simulink model "Mip_Balance_Demo_Multi_Rate"  (R2018b)
settings: Solver=FixedStepAuto  StartTime=0.0  StopTime=inf  RelTol=1e-3
undefined symbols (not defined in the file): DiscIntNeverNeededParam
libraries: simulink x2, bbblueSensorLib x2, bbblueActuatorLib x2, bbblueBasicLib x2, simulink_extras x1
settings Model: SimulationMode=external  Creator=ktalke  LastModifiedBy=ktalke
settings SolverCC: PositivePriorityOrder=on  AutoInsertRateTranBlk=on
settings OptimizationCC: EnhancedBackFolding=on  PassReuseOutputArgsAs=Individual arguments  MaxStackSize=64  OptimizeBlockOrder=speed  DifferentSizesBufferReuse=on  OptimizationCustomize=off
settings DebuggingCC: ParameterTunabilityLossMsg=error  LibraryContextMissingDiagnostic=none
settings HardwareCC: ProdBitPerPointer=32  ProdBitPerSizeT=32  ProdBitPerPtrDiffT=32  ProdLargestAtomicInteger=Long  ProdLargestAtomicFloat=Double  ProdWordSize=32  ProdHWDeviceType=ARM Compatible->ARM Cortex
settings SFSimCC: SimUseLocalCustomCode=off  MATLABDynamicMemAlloc=off
settings RTWCC: SystemTargetFile=ert.tlc  HardwareBoard=BeagleBone Blue  TLCOptions="-aInlineSetEventsForThisBaseRateFcn=TLC_FALSE -aSuppressMultiTaskScheduler=TLC_FALSE  -aRateBasedStepFcn=0"  TemplateMakefile=ert_default_tmf  RTWUseLocalCustomCode=off  Toolchain=GNU GCC BeagleBone Blue  IncludeHyperlinkInReport=on
settings CodeAppCC: ForceParamTrailComments=on  IgnoreCustomStorageClasses=off  OperatorAnnotations=on  SimulinkDataObjDesc=on  SFDataObjDesc=on  InsertBlockDesc=on
settings ERTTargetCC: SupportVariableSizeSignals=on

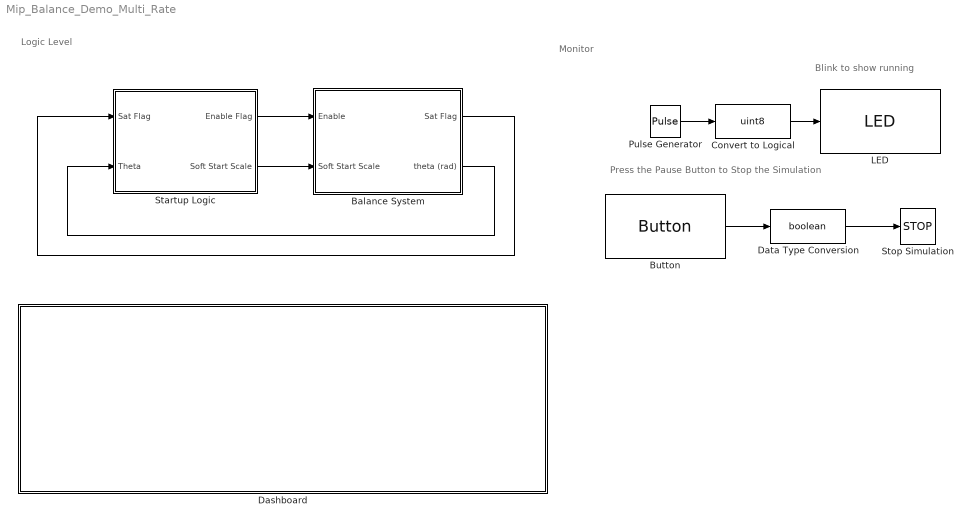
== system Mip_Balance_Demo_Multi_Rate ==
  note: Press the Pause Button to Stop the Simulation
  note: Logic Level
  note: Monitor
  note: Blink to show running
  Balance System : Subsystem  TreatAsAtomicUnit=on
  Button : bbblueBasicLib/Button  Button=Pause  SampleTime=0.1  SimulateUsing=Code generation
      settings: SourceProductName=Simulink Coder Support Package for BeagleBone Blue Hardware
  Convert to Logical : DataTypeConversion  OutDataTypeStr=uint8
  Dashboard : Subsystem
  Data Type Conversion : DataTypeConversion  OutDataTypeStr=boolean
  LED : bbblueBasicLib/LED  LED=Green
      settings: SourceProductName=Simulink Coder Support Package for BeagleBone Blue Hardware
  Pulse Generator : DiscretePulseGenerator  Period=10  PulseWidth=5  SampleTime=0.1
  Startup Logic : Subsystem
  Stop Simulation : Stop
  wires:
  Button/1 -> Data Type Conversion/1
  Startup Logic/2(Soft Start Scale) -> Balance System/2(Soft Start Scale)
  Pulse Generator/1 -> Convert to Logical/1
  Balance System/1(Sat Flag) -> Startup Logic/1(Sat Flag)
  Balance System/2(theta (rad)) -> Startup Logic/2(Theta)
  Data Type Conversion/1 -> Stop Simulation/1
  Startup Logic/1(Enable Flag) -> Balance System/1(Enable)
  Convert to Logical/1 -> LED/1

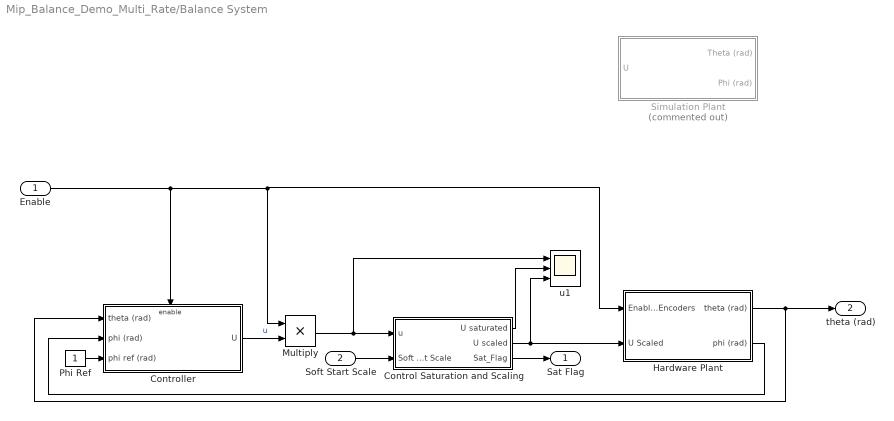
== system Mip_Balance_Demo_Multi_Rate/Balance System ==
  Enable : Inport
  Soft Start Scale : Inport  Port=2
  Control Saturation and Scaling : Subsystem
  Controller : Subsystem
  Hardware Plant : Subsystem
  Multiply : Product
  Phi Ref : Constant
  Simulation Plant : Subsystem  Commented=on
  u1 : Scope  NumInputPorts=3
  Sat Flag : Outport
  theta (rad) : Outport  Port=2
  wires:
  Phi Ref/1 -> Controller/3(phi ref (rad))
  Control Saturation and Scaling/1(U saturated) -> u1/2
  Control Saturation and Scaling/2(U scaled) -> Hardware Plant/2(U Scaled), u1/3
  Control Saturation and Scaling/3(Sat_Flag) -> Sat Flag/1
  Soft Start Scale/1 -> Control Saturation and Scaling/2(Soft Start Scale)
  Enable/1 -> Controller/Enable, Hardware Plant/1(Enable Encoders), Multiply/1
  Hardware Plant/1(theta (rad)) -> Controller/1(theta (rad)), theta (rad)/1
  Controller/1(U) -> Multiply/2  "u"
  Multiply/1 -> u1/1, Control Saturation and Scaling/1(u)
  Hardware Plant/2(phi (rad)) -> Controller/2(phi (rad))

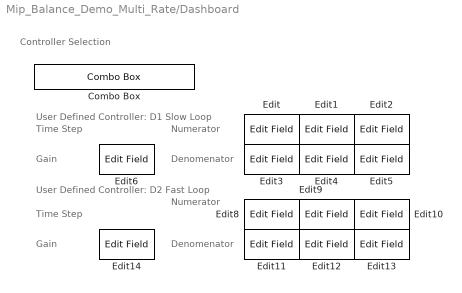
== system Mip_Balance_Demo_Multi_Rate/Dashboard ==
  note: Time Step
  note: Gain
  note: User Defined Controller: D1 Slow Loop
  note: Numerator
  note: Controller Selection
  note: Denomenator
  note: Numerator
  note: Denomenator
  note: Time Step
  note: User Defined Controller: D2 Fast Loop
  note: Gain
  Combo Box : ComboBox  WebBlockId=279  LabelPosition=Hide  SelectedLabel=200hz/20hz
      settings: Values={{'200 hz/200hz', '100hz/100hz', '100hz/50hz', '200hz/20hz', 'User Defined'}, [0 1 2 3 4]}
  Edit : EditField  WebBlockId=307  LabelPosition=Hide  ShowInitialText=on  Alignment=Center
  Edit1 : EditField  WebBlockId=313  LabelPosition=Hide  ShowInitialText=on  Alignment=Center
  Edit10 : EditField  WebBlockId=353  LabelPosition=Hide  ShowInitialText=on  Alignment=Center
  Edit11 : EditField  WebBlockId=354  LabelPosition=Hide  ShowInitialText=on  Alignment=Center
  Edit12 : EditField  WebBlockId=355  LabelPosition=Hide  ShowInitialText=on  Alignment=Center
  Edit13 : EditField  WebBlockId=356  LabelPosition=Hide  ShowInitialText=on  Alignment=Center
  Edit14 : EditField  WebBlockId=357  LabelPosition=Hide  ShowInitialText=on  Alignment=Center
  Edit2 : EditField  WebBlockId=314  LabelPosition=Hide  ShowInitialText=on  Alignment=Center
  Edit3 : EditField  WebBlockId=315  LabelPosition=Hide  ShowInitialText=on  Alignment=Center
  Edit4 : EditField  WebBlockId=316  LabelPosition=Hide  ShowInitialText=on  Alignment=Center
  Edit5 : EditField  WebBlockId=317  LabelPosition=Hide  ShowInitialText=on  Alignment=Center
  Edit6 : EditField  WebBlockId=337  LabelPosition=Hide  ShowInitialText=on  Alignment=Center
  Edit8 : EditField  WebBlockId=351  LabelPosition=Hide  ShowInitialText=on  Alignment=Center
  Edit9 : EditField  WebBlockId=352  LabelPosition=Hide  ShowInitialText=on  Alignment=Center

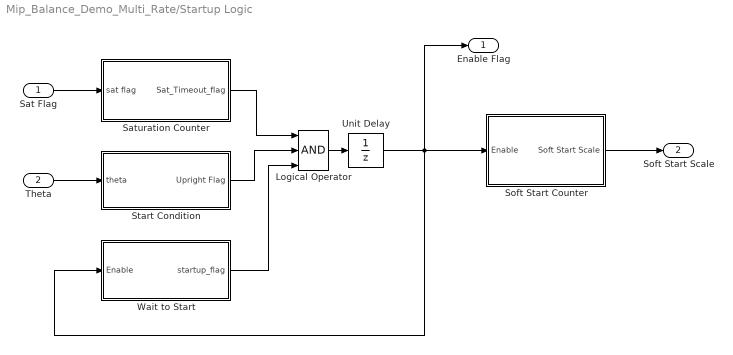
== system Mip_Balance_Demo_Multi_Rate/Startup Logic ==
  Sat Flag : Inport
  Theta : Inport  Port=2
  Logical Operator : Logic  Inputs=3  AllPortsSameDT=off  OutDataTypeStr=boolean
  Saturation Counter : Subsystem
  "Soft Start Counter " : Subsystem
  Start Condition : Subsystem
  Unit Delay : UnitDelay  SampleTime=-1
  Wait to Start : Subsystem
  Enable Flag : Outport
  Soft Start Scale : Outport  Port=2
  wires:
  Wait to Start/1(startup_flag) -> Logical Operator/3
  Logical Operator/1 -> Unit Delay/1
  Start Condition/1(Upright Flag) -> Logical Operator/2
  Saturation Counter/1(Sat_Timeout_flag) -> Logical Operator/1
  "Soft Start Counter "/1(Soft Start Scale) -> Soft Start Scale/1
  Sat Flag/1 -> Saturation Counter/1(sat flag)
  Theta/1 -> Start Condition/1(theta)
  Unit Delay/1 -> Enable Flag/1, "Soft Start Counter "/1(Enable), Wait to Start/1(Enable)

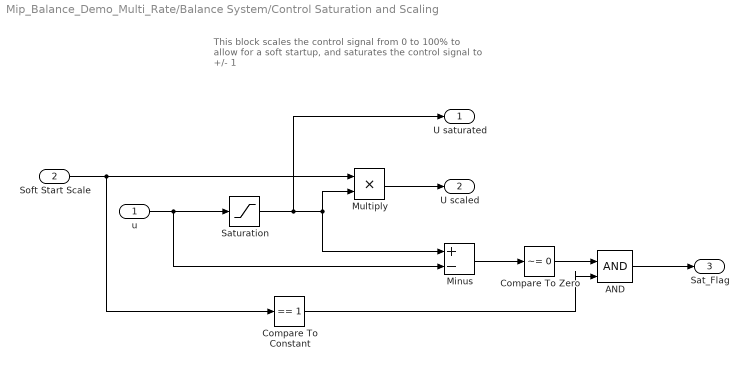
== system Mip_Balance_Demo_Multi_Rate/Balance System/Control Saturation and Scaling ==
  note: This block scales the control signal from 0 to 100% to allow for a soft startup, and saturates the control signal to +/- 1
  u : Inport
  Soft Start Scale : Inport  Port=2
  AND : Logic  IconShape=distinctive  AllPortsSameDT=off  OutDataTypeStr=boolean
  Compare To Constant : simulink/Logic and Bit Operations/Compare To Constant  relop===  const=1  OutDataTypeStr=boolean
  Compare To Zero : simulink/Logic and Bit Operations/Compare To Zero  relop=~=  OutDataTypeStr=boolean
  Minus : Sum  Inputs=+-
  Multiply : Product
  Saturation : Saturate  UpperLimit=1  LowerLimit=-1
  U saturated : Outport
  U scaled : Outport  Port=2  OutDataTypeStr=double  PortDimensions=[1 1]  SampleTime=[0.01,0]
  Sat_Flag : Outport  Port=3
  wires:
  u/1 -> Minus/2, Saturation/1
  Minus/1 -> Compare To Zero/1
  Soft Start Scale/1 -> Compare To Constant/1, Multiply/1
  Multiply/1 -> U scaled/1
  Saturation/1 -> U saturated/1, Minus/1, Multiply/2
  Compare To Zero/1 -> AND/1
  Compare To Constant/1 -> AND/2
  AND/1 -> Sat_Flag/1

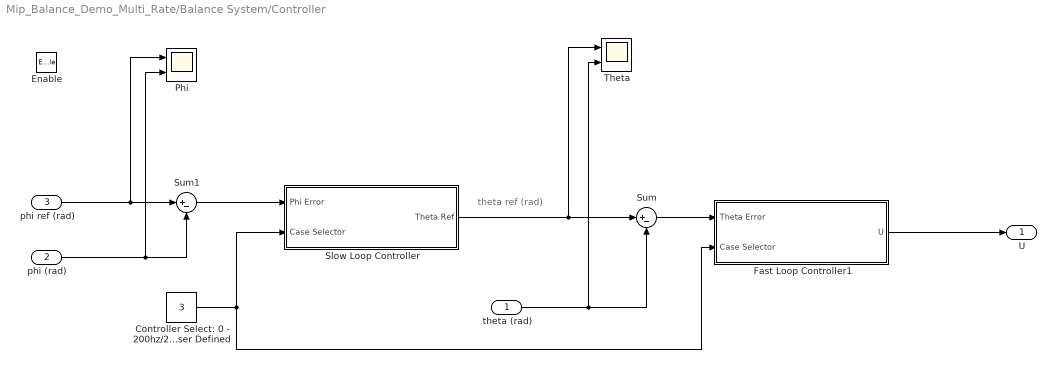
== system Mip_Balance_Demo_Multi_Rate/Balance System/Controller ==
  note: theta ref (rad)
  theta (rad) : Inport
  phi (rad) : Inport  Port=2
  phi ref (rad) : Inport  Port=3
  Enable : EnablePort  StatesWhenEnabling=reset  PropagateVarSize=During execution
  Controller Select: 0 - 200hz/200hz 1 - 100hz/100hz 2 - 100hz/50hz 3 - 200hz/20hz 4 - User Defined : Constant  Value=3
  Fast Loop Controller1 : Subsystem
  Phi : Scope  NumInputPorts=2
  Slow Loop Controller : Subsystem
  Sum : Sum  Inputs=|+-
  Sum1 : Sum  Inputs=|+-
  Theta : Scope  NumInputPorts=2
  U : Outport
  wires:
  phi ref (rad)/1 -> Phi/1, Sum1/1
  theta (rad)/1 -> Theta/2, Sum/2
  phi (rad)/1 -> Sum1/2, Phi/2
  Sum1/1 -> Slow Loop Controller/1(Phi Error)
  Slow Loop Controller/1(Theta Ref) -> Theta/1, Sum/1
  Controller Select: 0 - 200hz/200hz 1 - 100hz/100hz 2 - 100hz/50hz 3 - 200hz/20hz 4 - User Defined/1 -> Fast Loop Controller1/2(Case Selector), Slow Loop Controller/2(Case Selector)
  Sum/1 -> Fast Loop Controller1/1(Theta Error)
  Fast Loop Controller1/1(U) -> U/1

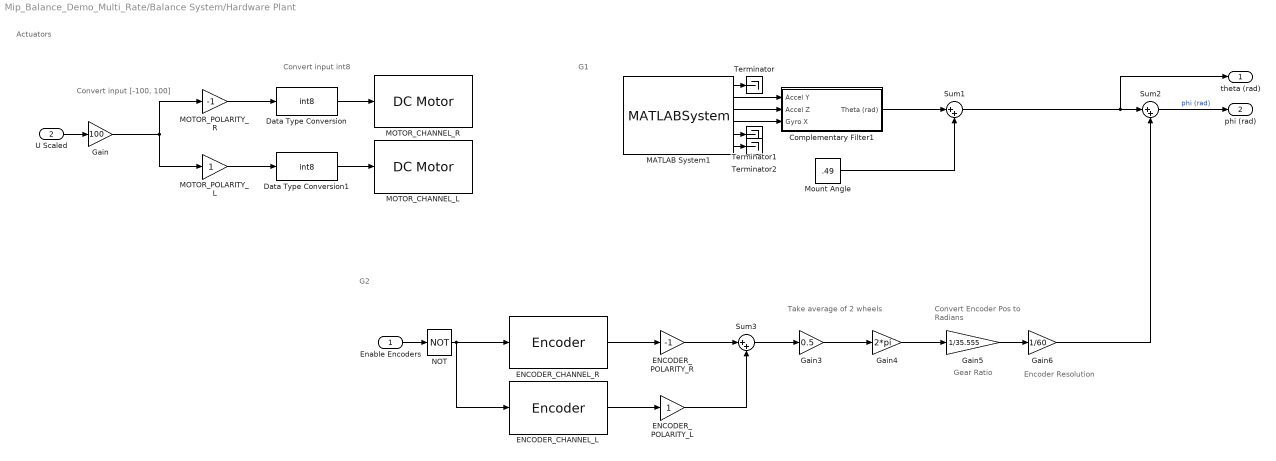
== system Mip_Balance_Demo_Multi_Rate/Balance System/Hardware Plant ==
  note: G2
  note: G1
  note: Actuators
  note: Convert input
      | [-100, 100]
  note: Convert input
      | int8
  note: Gear Ratio
  note: Encoder
      | Resolution
  note: Convert Encoder Pos
      | to Radians
  note: Take average
      | of 2 wheels
  Enable Encoders : Inport
  U Scaled : Inport  Port=2
  Complementary Filter1 : Subsystem
  Data Type Conversion : DataTypeConversion  OutDataTypeStr=int8  SaturateOnIntegerOverflow=on  RndMeth=Zero
  Data Type Conversion1 : DataTypeConversion  OutDataTypeStr=int8  SaturateOnIntegerOverflow=on  RndMeth=Zero
  ENCODER_CHANNEL_L : bbblueSensorLib/Encoder  Channel=3  Mode=Reset by external signal  SampleTime=0.005  SimulateUsing=Code generation
      settings: SourceProductName=Simulink Coder Support Package for BeagleBone Blue Hardware
  ENCODER_CHANNEL_R : bbblueSensorLib/Encoder  Channel=2  Mode=Reset by external signal  SampleTime=0.005  SimulateUsing=Code generation
      settings: SourceProductName=Simulink Coder Support Package for BeagleBone Blue Hardware
  ENCODER_POLARITY_L : Gain
  ENCODER_POLARITY_R : Gain  Gain=-1
  Gain : Gain  Gain=100
  Gain3 : Gain  Gain=0.5  OutDataTypeStr=double
  Gain4 : Gain  Gain=2*pi
  Gain5 : Gain  Gain=1/35.555
  Gain6 : Gain  Gain=1/60
  MATLAB System1 : MATLABSystem  System=beagleboneblue.fccr_bbblueIMU  SampleTime=0.005
      mask Type: beagleboneblue.fccr_bbblueIMU
      mask Display:
      | color('white');
      | plot([100,100,100,100]*1,[100,100,100,100]*1);
      | plot([100,100,100,100]*0,[100,100,100,100]*0);
      | color('blue');
      | text(100, 92, ' BB BLUE ', 'horizontalAlignment', 'right');
      | color('black');
      | text(52,52,' IMU','horizontalAlignment','center');
      | color('black');
  MOTOR_CHANNEL_L : bbblueActuatorLib/DC Motor  index=3  stopaction=Free Spin  SimulateUsing=Code generation
      settings: SourceProductName=Simulink Coder Support Package for BeagleBone Blue Hardware
  MOTOR_CHANNEL_R : bbblueActuatorLib/DC Motor  index=2  stopaction=Free Spin  SimulateUsing=Code generation
      settings: SourceProductName=Simulink Coder Support Package for BeagleBone Blue Hardware
  MOTOR_POLARITY_L : Gain
  MOTOR_POLARITY_R : Gain  Gain=-1
  Mount Angle : Constant  Value=.49
  NOT : Logic  Operator=NOT  IconShape=distinctive  AllPortsSameDT=off  OutDataTypeStr=boolean
  Sum1 : Sum  Inputs=|++
  Sum2 : Sum  Inputs=|++
  Sum3 : Sum  Inputs=|++
  Terminator : Terminator
  Terminator1 : Terminator
  Terminator2 : Terminator
  theta (rad) : Outport
  phi (rad) : Outport  Port=2
  wires:
  Sum2/1 -> phi (rad)/1  "phi (rad)"
  Gain6/1 -> Sum2/2
  Data Type Conversion1/1 -> MOTOR_CHANNEL_L/1
  MOTOR_POLARITY_R/1 -> Data Type Conversion/1
  Data Type Conversion/1 -> MOTOR_CHANNEL_R/1
  U Scaled/1 -> Gain/1
  MOTOR_POLARITY_L/1 -> Data Type Conversion1/1
  Gain/1 -> MOTOR_POLARITY_R/1, MOTOR_POLARITY_L/1
  Sum1/1 -> theta (rad)/1, Sum2/1
  MATLAB System1/1 -> Terminator/1
  Mount Angle/1 -> Sum1/2
  MATLAB System1/6 -> Terminator2/1
  Complementary Filter1/1(Theta (rad)) -> Sum1/1
  MATLAB System1/5 -> Terminator1/1
  Enable Encoders/1 -> NOT/1
  Gain5/1 -> Gain6/1
  ENCODER_CHANNEL_R/1 -> ENCODER_POLARITY_R/1
  Sum3/1 -> Gain3/1
  ENCODER_POLARITY_R/1 -> Sum3/1
  NOT/1 -> ENCODER_CHANNEL_L/1, ENCODER_CHANNEL_R/1
  Gain4/1 -> Gain5/1
  ENCODER_CHANNEL_L/1 -> ENCODER_POLARITY_L/1
  ENCODER_POLARITY_L/1 -> Sum3/2
  Gain3/1 -> Gain4/1
  MATLAB System1/2 -> Complementary Filter1/1(Accel Y)
  MATLAB System1/3 -> Complementary Filter1/2(Accel Z)
  MATLAB System1/4 -> Complementary Filter1/3(Gyro X)

== system Mip_Balance_Demo_Multi_Rate/Balance System/Simulation Plant ==
  U : Inport
  G1 Transfer Function : TransferFcn  Numerator=-420.4  Denominator=[1 12.1 088.24 -963.6]
  G2 Transfer Function : TransferFcn  Numerator=[-0.0002636 0 113.4]  Denominator=[1 0 0]
  Theta (rad) : Outport
  Phi (rad) : Outport  Port=2
  wires:
  G2 Transfer Function/1 -> Phi (rad)/1
  U/1 -> G1 Transfer Function/1
  G1 Transfer Function/1 -> G2 Transfer Function/1, Theta (rad)/1

== system Mip_Balance_Demo_Multi_Rate/Startup Logic/Saturation Counter ==
  note: Saturation Detection Threshold:
      | This block checks how long the motor has been saturated, and generates a disable flag
  sat flag : Inport
  Discrete-Time Integrator : DiscreteIntegrator  ExternalReset=falling  SampleTime=-1  ICPrevOutput=DiscIntNeverNeededParam  ICPrevScaledInput=DiscIntNeverNeededParam
  Relational Operator : RelationalOperator  Operator=<  OutDataTypeStr=boolean  RndMeth=Simplest
  Sat Timeout : Constant  Value=.5
  Sat_Timeout_flag : Outport
  wires:
  Relational Operator/1 -> Sat_Timeout_flag/1
  Sat Timeout/1 -> Relational Operator/2
  Discrete-Time Integrator/1 -> Relational Operator/1
  sat flag/1 -> Discrete-Time Integrator/1, Discrete-Time Integrator/2

== system Mip_Balance_Demo_Multi_Rate/Startup Logic/Soft Start Counter  ==
  note: Soft Start Detection Threshold:
      | This block generates a signal to scale up the input from 0 to 100% for the specified soft start time
  Enable : Inport
  Data Type Conversion : DataTypeConversion  OutDataTypeStr=double
  Discrete-Time Integrator : DiscreteIntegrator  ExternalReset=rising  SampleTime=-1  ICPrevOutput=DiscIntNeverNeededParam  ICPrevScaledInput=DiscIntNeverNeededParam
  Limits : Product  Inputs=*/
  Saturation : Saturate  UpperLimit=1  LowerLimit=0
  Soft Start Time1 : Constant  Value=.9
  Soft Start Scale : Outport
  wires:
  Limits/1 -> Saturation/1
  Discrete-Time Integrator/1 -> Limits/1
  Soft Start Time1/1 -> Limits/2
  Enable/1 -> Data Type Conversion/1, Discrete-Time Integrator/2
  Saturation/1 -> Soft Start Scale/1
  Data Type Conversion/1 -> Discrete-Time Integrator/1

== system Mip_Balance_Demo_Multi_Rate/Startup Logic/Start Condition ==
  note: Upright Detection Threshold:
      | This block checks the angle theta to see if it near the stability point, and produces an enable flag
  theta : Inport
  Abs : Abs
  Relational Operator : RelationalOperator  OutDataTypeStr=boolean  RndMeth=Simplest
  Relational Operator1 : RelationalOperator  Operator=<  OutDataTypeStr=boolean  RndMeth=Simplest
  Start Angle : Constant  Value=.6
  Start Counter : DiscreteIntegrator  ExternalReset=falling  SampleTime=-1  RndMeth=Zero  SaturateOnIntegerOverflow=on  UpperSaturationLimit=100  LowerSaturationLimit=-100  ICPrevOutput=DiscIntNeverNeededParam  ICPrevScaledInput=DiscIntNeverNeededParam
  Start Timeout : Constant
  Upright Flag : Outport
  wires:
  theta/1 -> Abs/1
  Start Counter/1 -> Relational Operator/1
  Relational Operator/1 -> Upright Flag/1
  Abs/1 -> Relational Operator1/1
  Start Timeout/1 -> Relational Operator/2
  Relational Operator1/1 -> Start Counter/2, Start Counter/1
  Start Angle/1 -> Relational Operator1/2

== system Mip_Balance_Demo_Multi_Rate/Startup Logic/Wait to Start ==
  note: Startup Detection Threshold:
      | This block enforces a wait time before allowing any control to start. The purpose is to allow the complementary filter time to stabilize, and to give a break if any other disable flag was triggered.
  Enable : Inport
  Constant : Constant
  Relational Operator : RelationalOperator  OutDataTypeStr=boolean  RndMeth=Simplest
  Wait Counter : DiscreteIntegrator  ExternalReset=falling  SampleTime=-1  SaturateOnIntegerOverflow=on  ICPrevOutput=DiscIntNeverNeededParam  ICPrevScaledInput=DiscIntNeverNeededParam
  Wait to Start : Constant  Value=3
  startup_flag : Outport
  wires:
  Wait Counter/1 -> Relational Operator/1
  Constant/1 -> Wait Counter/1
  Wait to Start/1 -> Relational Operator/2
  Relational Operator/1 -> startup_flag/1
  Enable/1 -> Wait Counter/2

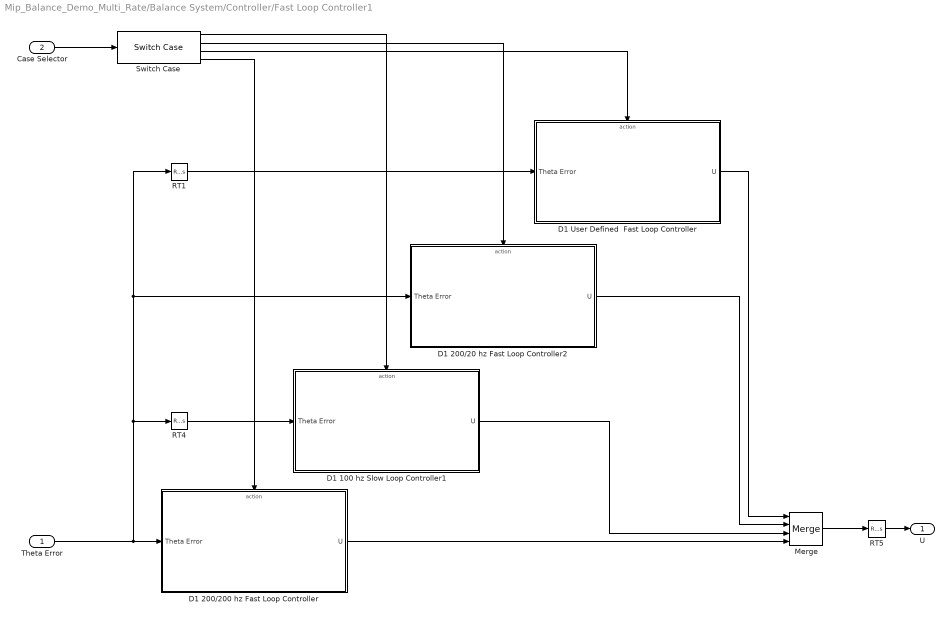
== system Mip_Balance_Demo_Multi_Rate/Balance System/Controller/Fast Loop Controller1 ==
  Theta Error : Inport
  Case Selector : Inport  Port=2
  D1 100 hz Slow Loop Controller1 : Subsystem  TreatAsAtomicUnit=on
  D1 200/20 hz Fast Loop Controller2 : Subsystem  TreatAsAtomicUnit=on
  D1 200/200 hz Fast Loop Controller : Subsystem  TreatAsAtomicUnit=on
  D1 User Defined  Fast Loop Controller : Subsystem  TreatAsAtomicUnit=on
  Merge : Merge  Inputs=4
  RT1 : RateTransition  OutPortSampleTime=0.005
  RT4 : RateTransition  OutPortSampleTime=0.01
  RT5 : RateTransition  OutPortSampleTime=0.005
  Switch Case : SwitchCase  CaseConditions={[1,2],3,4}
  U : Outport
  wires:
  Case Selector/1 -> Switch Case/1
  Theta Error/1 -> RT4/1, RT1/1, D1 200/20 hz Fast Loop Controller2/1(Theta Error), D1 200/200 hz Fast Loop Controller/1(Theta Error)
  Switch Case/4 -> D1 200/200 hz Fast Loop Controller/Action
  RT4/1 -> D1 100 hz Slow Loop Controller1/1(Theta Error)
  Merge/1 -> RT5/1
  RT5/1 -> U/1
  Switch Case/1 -> D1 100 hz Slow Loop Controller1/Action
  Switch Case/2 -> D1 200/20 hz Fast Loop Controller2/Action
  RT1/1 -> D1 User Defined  Fast Loop Controller/1(Theta Error)
  D1 User Defined  Fast Loop Controller/1(U) -> Merge/1
  D1 200/20 hz Fast Loop Controller2/1(U) -> Merge/2
  D1 100 hz Slow Loop Controller1/1(U) -> Merge/3
  D1 200/200 hz Fast Loop Controller/1(U) -> Merge/4
  Switch Case/3 -> D1 User Defined  Fast Loop Controller/Action

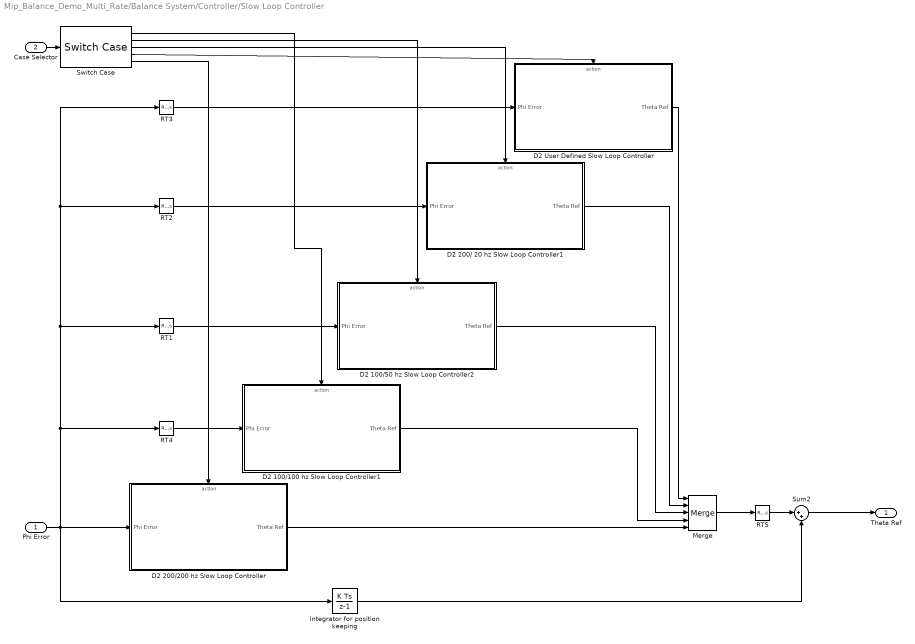
== system Mip_Balance_Demo_Multi_Rate/Balance System/Controller/Slow Loop Controller ==
  Phi Error : Inport
  Case Selector : Inport  Port=2
  D2 100/100 hz Slow Loop Controller1 : Subsystem  TreatAsAtomicUnit=on
  D2 100/50 hz Slow Loop Controller2 : Subsystem  TreatAsAtomicUnit=on
  "D2 200/ 20 hz Slow Loop Controller1 " : Subsystem  TreatAsAtomicUnit=on
  D2 200/200 hz Slow Loop Controller : Subsystem  TreatAsAtomicUnit=on
  D2 User Defined Slow Loop Controller : Subsystem  TreatAsAtomicUnit=on
  Integrator for position keeping : DiscreteIntegrator  gainval=.005  SampleTime=-1  ICPrevOutput=DiscIntNeverNeededParam  ICPrevScaledInput=DiscIntNeverNeededParam
  Merge : Merge  Inputs=5
  RT1 : RateTransition  OutPortSampleTime=0.02
  RT2 : RateTransition  OutPortSampleTime=0.05
  RT3 : RateTransition  OutPortSampleTimeMultiple=.1  OutPortSampleTime=0.01
  RT4 : RateTransition  OutPortSampleTime=0.01
  RT5 : RateTransition  OutPortSampleTime=0.005
  Sum2 : Sum  Inputs=|++
  Switch Case : SwitchCase  CaseConditions={1,2,3,4}
  Theta Ref : Outport
  wires:
  Case Selector/1 -> Switch Case/1
  Switch Case/5 -> D2 200/200 hz Slow Loop Controller/Action
  Switch Case/1 -> D2 100/100 hz Slow Loop Controller1/Action
  RT4/1 -> D2 100/100 hz Slow Loop Controller1/1(Phi Error)
  Merge/1 -> RT5/1
  Switch Case/2 -> D2 100/50 hz Slow Loop Controller2/Action
  Switch Case/3 -> "D2 200/ 20 hz Slow Loop Controller1 "/Action
  RT2/1 -> "D2 200/ 20 hz Slow Loop Controller1 "/1(Phi Error)
  RT1/1 -> D2 100/50 hz Slow Loop Controller2/1(Phi Error)
  Integrator for position keeping/1 -> Sum2/2
  Phi Error/1 -> Integrator for position keeping/1, RT3/1, RT2/1, RT1/1, RT4/1, D2 200/200 hz Slow Loop Controller/1(Phi Error)
  Sum2/1 -> Theta Ref/1
  RT5/1 -> Sum2/1
  D2 200/200 hz Slow Loop Controller/1(Theta Ref) -> Merge/5
  D2 100/100 hz Slow Loop Controller1/1(Theta Ref) -> Merge/4
  D2 100/50 hz Slow Loop Controller2/1(Theta Ref) -> Merge/3
  "D2 200/ 20 hz Slow Loop Controller1 "/1(Theta Ref) -> Merge/2
  RT3/1 -> D2 User Defined Slow Loop Controller/1(Phi Error)
  Switch Case/4 -> D2 User Defined Slow Loop Controller/Action
  D2 User Defined Slow Loop Controller/1(Theta Ref) -> Merge/1

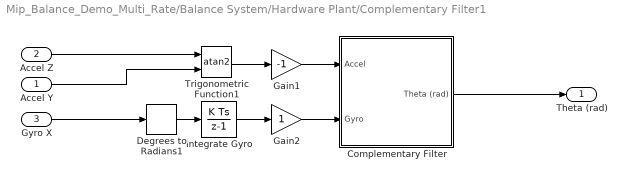
== system Mip_Balance_Demo_Multi_Rate/Balance System/Hardware Plant/Complementary Filter1 ==
  Accel Y : Inport
  Accel Z : Inport  Port=2
  Gyro X : Inport  Port=3
  Complementary Filter : Subsystem  mask(Complementary Filters){wc=.5, dt=.005}
      mask help:
      | dt - time step
      | wc - time constant
  Degrees to Radians1 : simulink_extras/Transformations/Degrees to Radians
  Gain1 : Gain  Gain=-1
  Gain2 : Gain
  Integrate Gyro : DiscreteIntegrator  SampleTime=-1  ICPrevOutput=DiscIntNeverNeededParam  ICPrevScaledInput=DiscIntNeverNeededParam
  Trigonometric Function1 : Trigonometry  Operator=atan2
  Theta (rad) : Outport
  wires:
  Complementary Filter/1(Theta (rad)) -> Theta (rad)/1
  Accel Z/1 -> Trigonometric Function1/1
  Gyro X/1 -> Degrees to Radians1/1
  Integrate Gyro/1 -> Gain2/1
  Degrees to Radians1/1 -> Integrate Gyro/1
  Accel Y/1 -> Trigonometric Function1/2
  Gain1/1 -> Complementary Filter/1(Accel)
  Trigonometric Function1/1 -> Gain1/1
  Gain2/1 -> Complementary Filter/2(Gyro)

== system Mip_Balance_Demo_Multi_Rate/Balance System/Controller/Fast Loop Controller1/D1 100 hz Slow Loop Controller1 ==
  Theta Error : Inport
  Action Port : ActionPort  ActionType=case
  D1 100hz Fast Loop Controller1 : DiscreteTransferFcn  Numerator=[-4.945, 8.862, -3.967]  Denominator=[1.000, -1.481, 0.4812]
  D1_GAIN1 : Gain  Gain=1.3
  U : Outport
  wires:
  D1 100hz Fast Loop Controller1/1 -> U/1
  D1_GAIN1/1 -> D1 100hz Fast Loop Controller1/1
  Theta Error/1 -> D1_GAIN1/1

== system Mip_Balance_Demo_Multi_Rate/Balance System/Controller/Fast Loop Controller1/D1 200//20 hz Fast Loop Controller2 ==
  Theta Error : Inport
  Action Port : ActionPort  ActionType=case
  D1 200hz/20hz Fast Loop Controller1 : DiscreteTransferFcn  Numerator=[-11.0745, 19.702, -8.7598]  Denominator=[1.000, -1.49756, 0.49756]
  D1_GAIN2 : Gain  Gain=.8
  U : Outport
  wires:
  D1 200hz/20hz Fast Loop Controller1/1 -> U/1
  D1_GAIN2/1 -> D1 200hz/20hz Fast Loop Controller1/1
  Theta Error/1 -> D1_GAIN2/1

== system Mip_Balance_Demo_Multi_Rate/Balance System/Controller/Fast Loop Controller1/D1 200//200 hz Fast Loop Controller ==
  Theta Error : Inport
  Action Port : ActionPort  ActionType=default
  D1 200hz/200hz Fast Loop Controller : DiscreteTransferFcn  Numerator=[-6.289, 11.91, -5.634]  Denominator=[1.000, -1.702, 0.7021]
  D1_GAIN : Gain  Gain=.8
  U : Outport
  wires:
  D1 200hz/200hz Fast Loop Controller/1 -> U/1
  D1_GAIN/1 -> D1 200hz/200hz Fast Loop Controller/1
  Theta Error/1 -> D1_GAIN/1

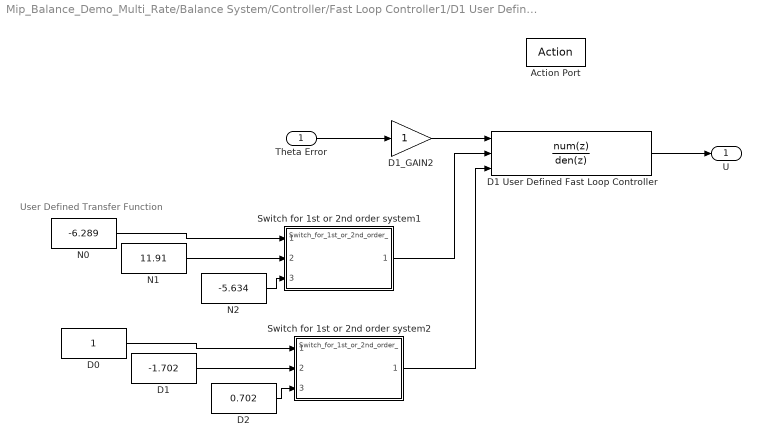
== system Mip_Balance_Demo_Multi_Rate/Balance System/Controller/Fast Loop Controller1/D1 User Defined  Fast Loop Controller ==
  note: User Defined Transfer Function
  Theta Error : Inport
  Action Port : ActionPort  ActionType=case
  D0 : Constant
  D1 : Constant  Value=-1.702
  D1 User Defined Fast Loop Controller : DiscreteTransferFcn  NumeratorSource=Input port  DenominatorSource=Input port  a0EqualsOne=on
      settings: InputPortMap=u0,p1,p3
  D1_GAIN2 : Gain
  D2 : Constant  Value=0.702
  N0 : Constant  Value=-6.289
  N1 : Constant  Value=11.91
  N2 : Constant  Value=-5.634
  Switch for 1st or 2nd order system1 : ModelReference  ModelNameDialog=Switch_for_1st_or_2nd_order_  SimulationMode=Normal  ModelReferenceVersion=1.140
  Switch for 1st or 2nd order system2 : ModelReference  ModelNameDialog=Switch_for_1st_or_2nd_order_  SimulationMode=Normal  ModelReferenceVersion=1.140
  U : Outport
  wires:
  D1 User Defined Fast Loop Controller/1 -> U/1
  D1_GAIN2/1 -> D1 User Defined Fast Loop Controller/1
  Theta Error/1 -> D1_GAIN2/1
  D2/1 -> Switch for 1st or 2nd order system2/3
  D0/1 -> Switch for 1st or 2nd order system2/1
  D1/1 -> Switch for 1st or 2nd order system2/2
  N0/1 -> Switch for 1st or 2nd order system1/1
  N2/1 -> Switch for 1st or 2nd order system1/3
  Switch for 1st or 2nd order system1/1 -> D1 User Defined Fast Loop Controller/2
  Switch for 1st or 2nd order system2/1 -> D1 User Defined Fast Loop Controller/3
  N1/1 -> Switch for 1st or 2nd order system1/2

== system Mip_Balance_Demo_Multi_Rate/Balance System/Controller/Slow Loop Controller/D2 100//100 hz Slow Loop Controller1 ==
  Phi Error : Inport
  Action Port : ActionPort  ActionType=case
  D2 100 hz Slow Loop Controller2 : DiscreteTransferFcn  Numerator="[0.28,  -0.5581,  0.2781]"  Denominator="[1.00000,  -1.86046,   0.86046]"
  D2_GAIN2 : Gain  Gain=.9
  Theta Ref : Outport
  wires:
  D2_GAIN2/1 -> D2 100 hz Slow Loop Controller2/1
  Phi Error/1 -> D2_GAIN2/1
  D2 100 hz Slow Loop Controller2/1 -> Theta Ref/1

== system Mip_Balance_Demo_Multi_Rate/Balance System/Controller/Slow Loop Controller/D2 100//50 hz Slow Loop Controller2 ==
  Phi Error : Inport
  Action Port : ActionPort  ActionType=case
  D2 50 hz SlowLoop Controller2 : DiscreteTransferFcn  Numerator="[0.2627,  -.5217, 0.259]"  Denominator="[1.00000,  -1.739, 0.7391]"
  D2_GAIN1 : Gain  Gain=.7
  Theta Ref : Outport
  wires:
  Phi Error/1 -> D2_GAIN1/1
  D2 50 hz SlowLoop Controller2/1 -> Theta Ref/1
  D2_GAIN1/1 -> D2 50 hz SlowLoop Controller2/1

== system Mip_Balance_Demo_Multi_Rate/Balance System/Controller/Slow Loop Controller/D2 200// 20 hz Slow Loop Controller1  ==
  Phi Error : Inport
  Action Port : ActionPort  ActionType=case
  D2 20 hz Slow Loop Controller2 : DiscreteTransferFcn  Numerator=[0.1636, -0.16289]  Denominator="[1.00000,  -.6326]"
  D2_GAIN3 : Gain  Gain=.7
  Theta Ref : Outport
  wires:
  D2 20 hz Slow Loop Controller2/1 -> Theta Ref/1
  D2_GAIN3/1 -> D2 20 hz Slow Loop Controller2/1
  Phi Error/1 -> D2_GAIN3/1

== system Mip_Balance_Demo_Multi_Rate/Balance System/Controller/Slow Loop Controller/D2 200//200 hz Slow Loop Controller ==
  Phi Error : Inport
  Action Port : ActionPort  ActionType=default
  D2 200 hz Slow Loop Controller1 : DiscreteTransferFcn  Numerator=[0.3858, -0.3858]  Denominator="[1.00000,  -.9277]"
  D2_GAIN : Gain  Gain=.7
  Theta Ref : Outport
  wires:
  D2 200 hz Slow Loop Controller1/1 -> Theta Ref/1
  Phi Error/1 -> D2_GAIN/1
  D2_GAIN/1 -> D2 200 hz Slow Loop Controller1/1

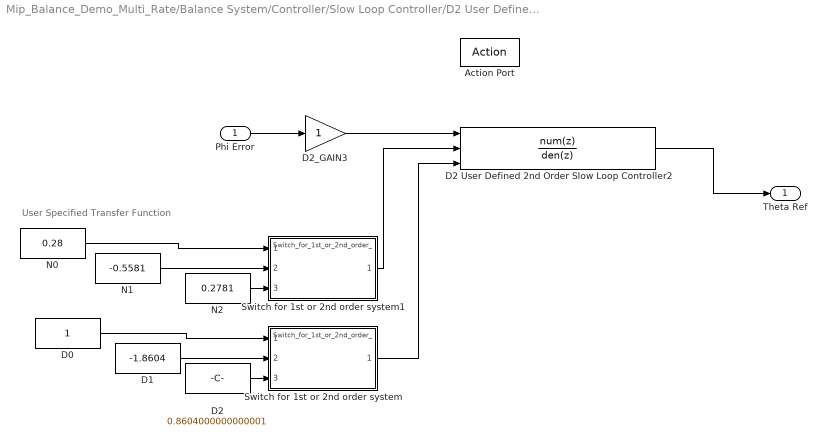
== system Mip_Balance_Demo_Multi_Rate/Balance System/Controller/Slow Loop Controller/D2 User Defined Slow Loop Controller ==
  note: User Specified Transfer Function
  Phi Error : Inport
  Action Port : ActionPort  ActionType=case
  D0 : Constant
  D1 : Constant  Value=-1.8604
  D2 : Constant  Value=0.8604000000000001
  D2 User Defined 2nd Order Slow Loop Controller2 : DiscreteTransferFcn  NumeratorSource=Input port  DenominatorSource=Input port  a0EqualsOne=on
      settings: InputPortMap=u0,p1,p3
  D2_GAIN3 : Gain
  N0 : Constant  Value=0.28
  N1 : Constant  Value=-0.5581
  N2 : Constant  Value=0.2781
  Switch for 1st or 2nd order system : ModelReference  ModelNameDialog=Switch_for_1st_or_2nd_order_  SimulationMode=Normal  ModelReferenceVersion=1.140
  Switch for 1st or 2nd order system1 : ModelReference  ModelNameDialog=Switch_for_1st_or_2nd_order_  SimulationMode=Normal  ModelReferenceVersion=1.140
  Theta Ref : Outport
  wires:
  D2_GAIN3/1 -> D2 User Defined 2nd Order Slow Loop Controller2/1
  Phi Error/1 -> D2_GAIN3/1
  N0/1 -> Switch for 1st or 2nd order system1/1
  D2 User Defined 2nd Order Slow Loop Controller2/1 -> Theta Ref/1
  Switch for 1st or 2nd order system1/1 -> D2 User Defined 2nd Order Slow Loop Controller2/2
  D0/1 -> Switch for 1st or 2nd order system/1
  D1/1 -> Switch for 1st or 2nd order system/2
  D2/1 -> Switch for 1st or 2nd order system/3
  Switch for 1st or 2nd order system/1 -> D2 User Defined 2nd Order Slow Loop Controller2/3
  N2/1 -> Switch for 1st or 2nd order system1/3
  N1/1 -> Switch for 1st or 2nd order system1/2

== system Mip_Balance_Demo_Multi_Rate/Balance System/Hardware Plant/Complementary Filter1/Complementary Filter ==
  Accel : Inport
  Gyro : Inport  Port=2
  "High Pass " : DiscreteTransferFcn  Numerator=[1 -1]  Denominator=[1 (wc*dt - 1)]
  "Low Pass " : DiscreteTransferFcn  Numerator=[0 wc*dt]  Denominator=[1 (wc*dt - 1)]
  Sum : Sum  Inputs=|++
  Theta (rad) : Outport
  wires:
  "High Pass "/1 -> Sum/2  "Theta (Gyro)"
  Accel/1 -> "Low Pass "/1
  Gyro/1 -> "High Pass "/1
  "Low Pass "/1 -> Sum/1  "Theta (Accel)"
  Sum/1 -> Theta (rad)/1
